simulink model "Excavator_Motion"  (R2026a)
settings: Solver=ode23t  StopTime=activeTestPos.getElement('swingAng').Time(end)  MaxStep=0.1  AbsTol=1e-3
PostLoadFcn:
  | set_param(bdroot,'IgnoredZcDiagnostic','none');
  | activeTestPos = ScenarioMotion.loadedBucketDigCycle;
model workspace: external: MAT-File ExcavatorAssemblyDataStruct.mat (data not in the file)
undefined symbols (not defined in the file or in its folder): Bo, Bu, gravity, materialWeight, P28Assembly, startDiggingZPos, velocityToYForceGain, X, Y, yForceMax, yForceToZForceGain, Z, zForceMax
libraries: sm_lib x79, nesl_utility x41, Excavator_Parts_Lib x8, simulink x2, simulink_extras x1
(part 1 of 3)
Description:
  | Excavator with Actuator Force Calculation
  | 
  | Copyright 2022-2026 The MathWorks, Inc.
settings Model: Creator=gabri  LastModifiedBy=smiller
settings SolverCC: MaxConsecutiveMinStep=10  ZeroCrossAlgorithm=Adaptive  DecoupledContinuousIntegration=on  MinimalZcImpactIntegration=on
settings DataIOCC: ExternalInput=activeTestPos  LoadExternalInput=on  SignalLoggingName=logsout_Excavator_Motion  ReturnWorkspaceOutputsName=simOut
settings DebuggingCC: IgnoredZcDiagnostic=none
settings SimscapeCC: SimscapeNominalValues="[{\"value\":\"1\",\"unit\":\"A\"},{\"value\":\"1\",\"unit\":\"bar\"},{\"value\":\"1\",\"unit\":\"cm^2\"},{\"value\":\"1\",\"unit\":\"cm^3/s\"},{\"value\":\"1\",\"unit\":\"kJ/kg\"},{\"value\":\"1\",\"unit\":\"kW\"},{\"value\":\"1\",\"unit\":\"l\"},{\"value\":\"1\",\"unit\":\"N\"},{\"value\":\"1\",\"unit\":\"N*m\"},{\"value\":\"1\",\"unit\":\"V\"}]"  SimscapeLogName=simlog_Excavator_Motion  SimscapeLogLimitData=off  SimscapeLogDataHistory=5000.0
settings DiagnosticsConfigSet: SimMechanicsConflictingReferenceFrames=none
settings ExplorerConfigSet: InternalSimMechanicsExplorerSettings="<ExplorerConfiguration><canonicalview>default</canonicalview><AnimationSetting><BasePlaybackSpeed>1.0</BasePlaybackSpeed><PlaybackSpeedFactor>1.0</PlaybackSpeedFactor></AnimationSetting><TilePanel><TileInfo><Tiles Columns=\"1\" Count=\"1\" Rows=\"1\"><Column Weight=\"1\"/><Row Weight=\"1\"/><Tile Height=\"1\" Width=\"1\" X=\"0\" Y=\"0\"/></Tiles></TileInfo><SceneInfo><SceneViewer><BGColor><R>1</R><G>1</G><B>1</B></BGColor><Camera><DoPerspective>off</DoPerspective><Position><X>27.5807103687801352</X><Y>37.4081583974126985</Y><Z>9.98244775872054291</Z></Position><Center><X>8.99598322856128263</X><Y>12.20284550619599</Y><Z>4.4342740611865441</Z></Center><Up><X>-0.106919570484384385</X><Y>-0.137906585416309235</Y><Z>0.984657290201138458</Z></Up><ViewLimDist>1</ViewLimDist><YLim>6.11731328526511131</YLim><XLim>12.9452235683135441</XLim></Camera></SceneViewer></SceneInfo></TilePanel><MechEditorPanel><Cameras/><GfxPanelCameraMap/><VideoCreator><PlaybackSpeedRatio>1.0</PlaybackSpeedRatio><FrameRate>30</FrameRate><VideoFormat>Motion JPEG AVI</VideoFormat><FrameSize>auto</FrameSize></VideoCreator></MechEditorPanel></ExplorerConfiguration>"

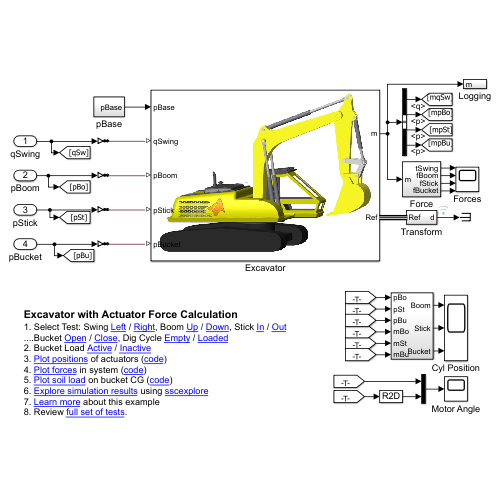
[thumbnail: Simulink's stored preview of the top-level diagram]
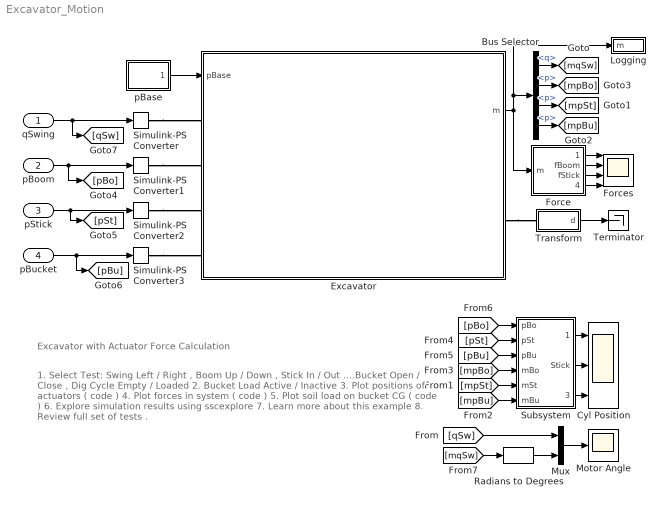
== system Excavator_Motion ==
  note: Excavator with Actuator Force Calculation
  note: 1. Select Test: Swing Left / Right , Boom Up / Down , Stick In / Out
      | ....Bucket Open / Close , Dig Cycle Empty / Loaded
      | 2. Bucket Load Active / Inactive
      | 3. Plot positions of actuators ( code )
      | 4. Plot forces in system ( code )
      | 5. Plot soil load on bucket CG ( code )
      | 6. Explore simulation results using sscexplore
      | 7. Learn more about this example
      | 8. Review full set of tests .
  qSwing : Inport
  pBoom : Inport  Port=2
  pStick : Inport  Port=3
  pBucket : Inport  Port=4
  Bus Selector : BusSelector  OutputSignals=Swing.q,Boom.p,Stick.p,Bucket.p
  Cyl Position : Scope  NumInputPorts=3
      settings: ActiveDisplayYMinimum=-0.10545  ActiveDisplayYMaximum=1.26585
  Excavator : Subsystem
      mask Display: image('Excavator_CAD_Full_IMAGE.png');
  Force : Subsystem
  Forces : Scope  NumInputPorts=4
      settings: ActiveDisplayYMinimum=-530.22843  ActiveDisplayYMaximum=1858.3528  DataLoggingVariableName=ScopeData2
  Logging : Subsystem
  Motor Angle : Scope
      settings: ActiveDisplayYMinimum=-135.21911  ActiveDisplayYMaximum=16.97108
  Mux : Mux  Inputs=2
  Radians to Degrees : simulink_extras/Transformations/Radians to Degrees
  Simulink-PS Converter : nesl_utility/Simulink-PS Converter  PhysicalDomain=network_engine_domain  SubClassName=ps_input  LeftPortType=input  RightPortType=output  PseudoPeriodic=off  Frequencies=[]  NoiseDistribution=none  NoiseParameters=[]  Unit=deg  AffineConversion=off  FilteringAndDerivatives=filter  SimscapeFilterOrder=2  InputFilterTimeConstant=0.05  UdotUserProvided=0
  Simulink-PS Converter1 : nesl_utility/Simulink-PS Converter  PhysicalDomain=network_engine_domain  SubClassName=ps_input  LeftPortType=input  RightPortType=output  PseudoPeriodic=off  Frequencies=[]  NoiseDistribution=none  NoiseParameters=[]  Unit=mm  AffineConversion=off  FilteringAndDerivatives=filter  SimscapeFilterOrder=2  InputFilterTimeConstant=0.05  UdotUserProvided=0
  Simulink-PS Converter2 : nesl_utility/Simulink-PS Converter  PhysicalDomain=network_engine_domain  SubClassName=ps_input  LeftPortType=input  RightPortType=output  PseudoPeriodic=off  Frequencies=[]  NoiseDistribution=none  NoiseParameters=[]  Unit=mm  AffineConversion=off  FilteringAndDerivatives=filter  SimscapeFilterOrder=2  InputFilterTimeConstant=0.05  UdotUserProvided=0
  Simulink-PS Converter3 : nesl_utility/Simulink-PS Converter  PhysicalDomain=network_engine_domain  SubClassName=ps_input  LeftPortType=input  RightPortType=output  PseudoPeriodic=off  Frequencies=[]  NoiseDistribution=none  NoiseParameters=[]  Unit=mm  AffineConversion=off  FilteringAndDerivatives=filter  SimscapeFilterOrder=2  InputFilterTimeConstant=0.05  UdotUserProvided=0
  Subsystem : Subsystem
  Terminator : Terminator
  Transform : Subsystem
  pBase : Subsystem
  wires:
  pBoom/1 -> Simulink-PS Converter1/1, [pBo]
  pStick/1 -> Simulink-PS Converter2/1, [pSt]
  qSwing/1 -> [qSw], Simulink-PS Converter/1
  pBucket/1 -> [pBu], Simulink-PS Converter3/1
  Excavator/1(m) -> Bus Selector/1, Logging/1(m), Force/1(m)
  Bus Selector/1 -> [mqSw]  "<q>"
  Bus Selector/2 -> [mpBo]  "<p>"
  Bus Selector/3 -> [mpSt]  "<p>"
  Bus Selector/4 -> [mpBu]  "<p>"
  [mpBo] -> Subsystem/4(mBo)
  [mpSt] -> Subsystem/5(mSt)
  [mpBu] -> Subsystem/6(mBu)
  Subsystem/1(Boom) -> Cyl Position/1
  Subsystem/2(Stick) -> Cyl Position/2
  Subsystem/3(Bucket) -> Cyl Position/3
  [pBo] -> Subsystem/1(pBo)
  [pSt] -> Subsystem/2(pSt)
  [pBu] -> Subsystem/3(pBu)
  [qSw] -> Mux/1
  [mqSw] -> Radians to Degrees/1
  Mux/1 -> Motor Angle/1
  Radians to Degrees/1 -> Mux/2
  Force/1(tSwing) -> Forces/1
  Force/2(fBoom) -> Forces/2
  Force/3(fStick) -> Forces/3
  Force/4(fBucket) -> Forces/4
  Transform/1(d) -> Terminator/1
  pBase/1(pBase) -> Excavator/1(pBase)
  connections:
  Simulink-PS Converter/RConn1 -- Excavator/LConn1
  Simulink-PS Converter1/RConn1 -- Excavator/LConn2
  Simulink-PS Converter2/RConn1 -- Excavator/LConn3
  Simulink-PS Converter3/RConn1 -- Excavator/LConn4
  Excavator/RConn1 -- Transform/LConn1

== system Excavator_Motion/Excavator ==
  pBase : Inport
  Machine : Subsystem
      mask Display: image('Excavator_CAD_Full_IMAGE.png');
  qSwing : PMIOPort  Side=Left
  pBoom : PMIOPort  Port=2  Side=Left
  pStick : PMIOPort  Port=3  Side=Left
  pBucket : PMIOPort  Port=4  Side=Left
  Ref : PMIOPort  Port=5  Side=Right
  m : Outport
  wires:
  Machine/1(m) -> m/1
  pBase/1 -> Machine/1(pBase)
  connections:
  qSwing/RConn1 -- Machine/LConn1
  pBoom/RConn1 -- Machine/LConn2
  pStick/RConn1 -- Machine/LConn3
  pBucket/RConn1 -- Machine/LConn4
  Machine/RConn1 -- Ref/RConn1

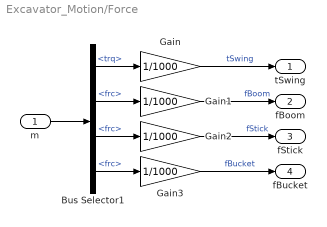
== system Excavator_Motion/Force ==
  m : Inport
  Bus Selector1 : BusSelector  OutputSignals=Swing.trq,Boom.frc,Stick.frc,Bucket.frc
  Gain{,1..3} (4 alike) : Gain  Gain=1/1000
  tSwing : Outport
  fBoom : Outport  Port=2
  fStick : Outport  Port=3
  fBucket : Outport  Port=4
  wires:
  Bus Selector1/1 -> Gain/1  "<trq>"
  Bus Selector1/2 -> Gain1/1  "<frc>"
  m/1 -> Bus Selector1/1
  Bus Selector1/3 -> Gain2/1  "<frc>"
  Bus Selector1/4 -> Gain3/1  "<frc>"
  Gain/1 -> tSwing/1  "tSwing"
  Gain1/1 -> fBoom/1  "fBoom"
  Gain2/1 -> fStick/1  "fStick"
  Gain3/1 -> fBucket/1  "fBucket"

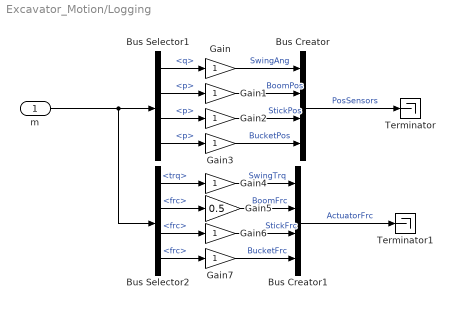
== system Excavator_Motion/Logging ==
  m : Inport
  Bus Creator : BusCreator  Inputs=4
  Bus Creator1 : BusCreator  Inputs=4
  Bus Selector1 : BusSelector  OutputSignals=Swing.q,Boom.p,Stick.p,Bucket.p
  Bus Selector2 : BusSelector  OutputSignals=Swing.trq,Boom.frc,Stick.frc,Bucket.frc
  Gain{,1..4,6..7} (7 alike) : Gain
  Gain5 : Gain  Gain=0.5
  Terminator : Terminator
  Terminator1 : Terminator
  wires:
  m/1 -> Bus Selector2/1, Bus Selector1/1
  Bus Selector1/1 -> Gain/1  "<q>"
  Bus Selector1/2 -> Gain1/1  "<p>"
  Bus Selector1/3 -> Gain2/1  "<p>"
  Bus Selector1/4 -> Gain3/1  "<p>"
  Gain/1 -> Bus Creator/1  "SwingAng"
  Gain1/1 -> Bus Creator/2  "BoomPos"
  Gain2/1 -> Bus Creator/3  "StickPos"
  Gain3/1 -> Bus Creator/4  "BucketPos"
  Bus Creator/1 -> Terminator/1  "PosSensors"
  Bus Selector2/4 -> Gain7/1  "<frc>"
  Bus Selector2/3 -> Gain6/1  "<frc>"
  Bus Selector2/2 -> Gain5/1  "<frc>"
  Bus Selector2/1 -> Gain4/1  "<trq>"
  Bus Creator1/1 -> Terminator1/1  "ActuatorFrc"
  Gain7/1 -> Bus Creator1/4  "BucketFrc"
  Gain6/1 -> Bus Creator1/3  "StickFrc"
  Gain5/1 -> Bus Creator1/2  "BoomFrc"
  Gain4/1 -> Bus Creator1/1  "SwingTrq"

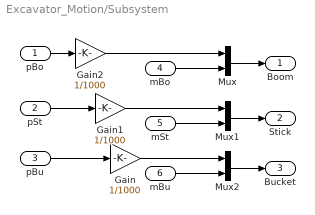
== system Excavator_Motion/Subsystem ==
  pBo : Inport
  pSt : Inport  Port=2
  pBu : Inport  Port=3
  mBo : Inport  Port=4
  mSt : Inport  Port=5
  mBu : Inport  Port=6
  Gain : Gain  Gain=1/1000
  Gain1 : Gain  Gain=1/1000
  Gain2 : Gain  Gain=1/1000
  Mux : Mux  Inputs=2
  Mux1 : Mux  Inputs=2
  Mux2 : Mux  Inputs=2
  Boom : Outport
  Stick : Outport  Port=2
  Bucket : Outport  Port=3
  wires:
  Mux1/1 -> Stick/1
  Mux/1 -> Boom/1
  Mux2/1 -> Bucket/1
  Gain/1 -> Mux2/1
  Gain2/1 -> Mux/1
  pBo/1 -> Gain2/1
  Gain1/1 -> Mux1/1
  pBu/1 -> Gain/1
  mBo/1 -> Mux/2
  pSt/1 -> Gain1/1
  mSt/1 -> Mux1/2
  mBu/1 -> Mux2/2

== system Excavator_Motion/Transform ==
  Part Pos Ori : Excavator_Parts_Lib/Part Pos Ori  SystemSampleTime=-1  VariantActivationTime=update diagram  EmptyChoice=off  PassThrough=off  PassThroughVariantControl=(default)  EmptyChoiceVariantControl=(default)  AllowFlexibleInterface=on  Latency=0  AutoFrameSizeCalculation=off
  Part Pos Ori1 : Excavator_Parts_Lib/Part Pos Ori  SystemSampleTime=-1  VariantActivationTime=update diagram  EmptyChoice=off  PassThrough=off  PassThroughVariantControl=(default)  EmptyChoiceVariantControl=(default)  AllowFlexibleInterface=on  Latency=0  AutoFrameSizeCalculation=off
  Simscape Bus : SimscapeBus  HierarchyStrings=Bo;Bu
  Ref : PMIOPort  Side=Left
  Out Bus Element : Outport  PortName=d  Element=Boom
  Out Bus Element1 : Outport  PortName=d  Element=Bucket
  wires:
  Part Pos Ori1/1 -> Out Bus Element/1
  Part Pos Ori/1 -> Out Bus Element1/1
  connections:
  Ref/RConn1 -- Simscape Bus/RConn1
  Part Pos Ori1/LConn1 -- Simscape Bus/LConn1
  Part Pos Ori/LConn1 -- Simscape Bus/LConn2

== system Excavator_Motion/pBase ==
  Bus Creator : BusCreator  Inputs=3
  Constant : Constant  Value=0
  Constant1 : Constant  Value=0
  Constant2 : Constant  Value=0
  pBase : Outport
  wires:
  Bus Creator/1 -> pBase/1
  Constant/1 -> Bus Creator/1  "px"
  Constant1/1 -> Bus Creator/2  "py"
  Constant2/1 -> Bus Creator/3  "qz"

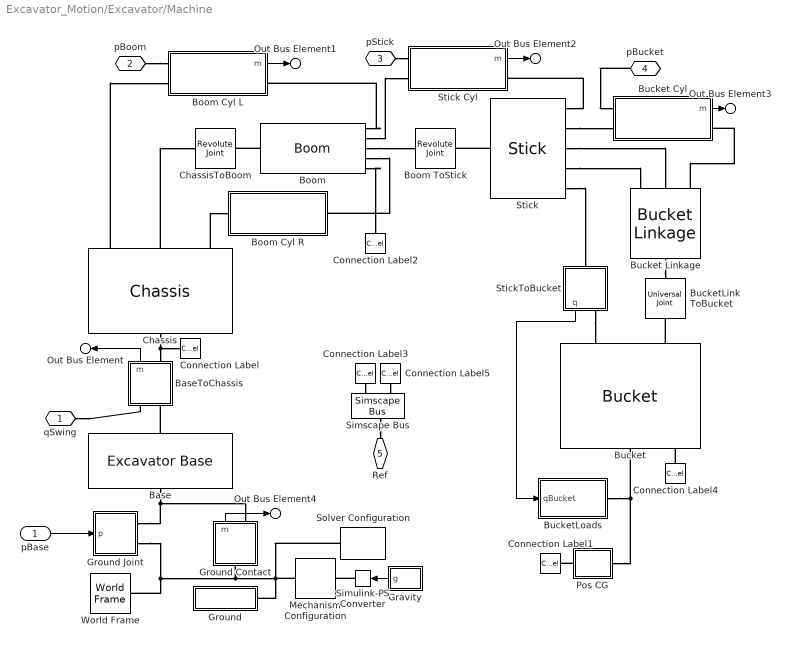
== system Excavator_Motion/Excavator/Machine ==
  pBase : Inport
  Base : Excavator_Parts_Lib/Excavator Base  Tag=AAA55596-1DB0-4345-9724-6685E48489E2
  BaseToChassis : Subsystem  Tag=1fdcb50d-bed1-4557-9df5-71c57fded59e
      mask Display: image('Excavator_Revolute_IMAGE.png')
  Boom : Excavator_Parts_Lib/Boom  Tag=FF941BC7-23B6-8A4E-AE2C-D7583C913694  opc=1  part_clr=excv_data.arm.clr
  Boom ToStick : sm_lib/Joints/Revolute Joint  JointMode=Normal  CompositeWrenchDir=FollowerOnBase  CompositeWrenchFrame=BaseFrame  SenseConstraintForce=off  SenseConstraintTorque=off  SenseTotalForce=off  SenseTotalTorque=off  PositionTargetSpecify=on  PositionTargetPriority=Low  PositionTargetValue=initBoomToStickRevPos  PositionTargetValueUnits=deg  VelocityTargetSpecify=off  VelocityTargetPriority=High  VelocityTargetValue=0  VelocityTargetValueUnits=deg/s  EquilibriumPosition=0  EquilibriumPositionUnits=deg  SpringStiffness=0  SpringStiffnessUnits=N*m/deg  DampingCoefficient=0  DampingCoefficientUnits=N*m/(deg/s)  LowerLimitSpecify=off  LowerLimitBound=-90  LowerLimitBoundUnits=deg  LowerLimitStiffness=1e4  LowerLimitStiffnessUnits=N*m/deg  LowerLimitDamping=10  LowerLimitDampingUnits=N*m/(deg/s)  LowerLimitTransitionRegionWidth=0.1  LowerLimitTransitionRegionWidthUnits=deg  UpperLimitSpecify=off  UpperLimitBound=90  UpperLimitBoundUnits=deg  UpperLimitStiffness=1e4  UpperLimitStiffnessUnits=N*m/deg  UpperLimitDamping=10  UpperLimitDampingUnits=N*m/(deg/s)  UpperLimitTransitionRegionWidth=0.1  UpperLimitTransitionRegionWidthUnits=deg  TorqueActuationMode=NoTorque  MotionActuationMode=ComputedMotion  SensePosition=off  SenseVelocity=off  SenseAcceleration=off  SenseTorqueForce=off  SenseLowerLimitTorqueForce=off  SenseUpperLimitTorqueForce=off
  Boom Cyl L : Subsystem
      mask Display: image('Excavator_Cylinder_Actuate_IMAGE.png')
  Boom Cyl R : Subsystem
      mask Display: image('Excavator_Cylinder_Actuate_IMAGE.png')
  Bucket : Excavator_Parts_Lib/Bucket  Tag=FF47B028-216B-7042-A7FD-934F60E6CEA6  opc=1  part_clr=excv_data.arm.clr
  Bucket Linkage : Excavator_Parts_Lib/Bucket Linkage
  Bucket Cyl : Subsystem
      mask Display: image('Excavator_Cylinder_Actuate_IMAGE.png')
  BucketLink ToBucket : sm_lib/Joints/Universal Joint  JointMode=Normal  CompositeWrenchDir=FollowerOnBase  CompositeWrenchFrame=BaseFrame  SenseConstraintForce=off  SenseConstraintTorque=off  SenseTotalForce=off  SenseTotalTorque=off  RxPositionTargetSpecify=on  RxPositionTargetPriority=Low  RxPositionTargetValue=-10  RxPositionTargetValueUnits=deg  RxVelocityTargetSpecify=off  RxVelocityTargetPriority=High  RxVelocityTargetValue=0  RxVelocityTargetValueUnits=deg/s  RxEquilibriumPosition=0  RxEquilibriumPositionUnits=deg  RxSpringStiffness=0  RxSpringStiffnessUnits=N*m/deg  RxDampingCoefficient=0  RxDampingCoefficientUnits=N*m/(deg/s)  RxLowerLimitSpecify=off  RxLowerLimitBound=-90  RxLowerLimitBoundUnits=deg  RxLowerLimitStiffness=1e4  RxLowerLimitStiffnessUnits=N*m/deg  RxLowerLimitDamping=10  RxLowerLimitDampingUnits=N*m/(deg/s)  RxLowerLimitTransitionRegionWidth=0.1  RxLowerLimitTransitionRegionWidthUnits=deg  RxUpperLimitSpecify=off  RxUpperLimitBound=90  RxUpperLimitBoundUnits=deg  RxUpperLimitStiffness=1e4  RxUpperLimitStiffnessUnits=N*m/deg  RxUpperLimitDamping=10  RxUpperLimitDampingUnits=N*m/(deg/s)  RxUpperLimitTransitionRegionWidth=0.1  RxUpperLimitTransitionRegionWidthUnits=deg  RxTorqueActuationMode=NoTorque  RxMotionActuationMode=ComputedMotion  RxSensePosition=off  RxSenseVelocity=off  RxSenseAcceleration=off  RxSenseTorqueForce=off  RxSenseLowerLimitTorqueForce=off  RxSenseUpperLimitTorqueForce=off  RyPositionTargetSpecify=on  RyPositionTargetPriority=High  RyPositionTargetValue=0  RyPositionTargetValueUnits=deg  RyVelocityTargetSpecify=off  RyVelocityTargetPriority=High  RyVelocityTargetValue=0  RyVelocityTargetValueUnits=deg/s  RyEquilibriumPosition=0  RyEquilibriumPositionUnits=deg  RySpringStiffness=0  RySpringStiffnessUnits=N*m/deg  RyDampingCoefficient=0  RyDampingCoefficientUnits=N*m/(deg/s)  RyLowerLimitSpecify=off  RyLowerLimitBound=-90  RyLowerLimitBoundUnits=deg  RyLowerLimitStiffness=1e4  RyLowerLimitStiffnessUnits=N*m/deg  RyLowerLimitDamping=10  RyLowerLimitDampingUnits=N*m/(deg/s)  RyLowerLimitTransitionRegionWidth=0.1  RyLowerLimitTransitionRegionWidthUnits=deg  RyUpperLimitSpecify=off  RyUpperLimitBound=90  RyUpperLimitBoundUnits=deg  RyUpperLimitStiffness=1e4  RyUpperLimitStiffnessUnits=N*m/deg  RyUpperLimitDamping=10  RyUpperLimitDampingUnits=N*m/(deg/s)  RyUpperLimitTransitionRegionWidth=0.1  RyUpperLimitTransitionRegionWidthUnits=deg  RyTorqueActuationMode=NoTorque  RyMotionActuationMode=ComputedMotion  RySensePosition=off  RySenseVelocity=off  RySenseAcceleration=off  RySenseTorqueForce=off  RySenseLowerLimitTorqueForce=off  RySenseUpperLimitTorqueForce=off
  BucketLoads : Subsystem
  Chassis : Excavator_Parts_Lib/Chassis  Tag=19F311DB-9E7A-8F4D-82CB-D8DCD5D4899B  opc=1
  ChassisToBoom : sm_lib/Joints/Revolute Joint  JointMode=Normal  CompositeWrenchDir=FollowerOnBase  CompositeWrenchFrame=BaseFrame  SenseConstraintForce=off  SenseConstraintTorque=off  SenseTotalForce=off  SenseTotalTorque=off  PositionTargetSpecify=on  PositionTargetPriority=Low  PositionTargetValue=initChassisToBoomRevPos  PositionTargetValueUnits=deg  VelocityTargetSpecify=off  VelocityTargetPriority=High  VelocityTargetValue=0  VelocityTargetValueUnits=deg/s  EquilibriumPosition=0  EquilibriumPositionUnits=deg  SpringStiffness=0  SpringStiffnessUnits=N*m/deg  DampingCoefficient=0  DampingCoefficientUnits=N*m/(deg/s)  LowerLimitSpecify=off  LowerLimitBound=-90  LowerLimitBoundUnits=deg  LowerLimitStiffness=1e4  LowerLimitStiffnessUnits=N*m/deg  LowerLimitDamping=10  LowerLimitDampingUnits=N*m/(deg/s)  LowerLimitTransitionRegionWidth=0.1  LowerLimitTransitionRegionWidthUnits=deg  UpperLimitSpecify=off  UpperLimitBound=90  UpperLimitBoundUnits=deg  UpperLimitStiffness=1e4  UpperLimitStiffnessUnits=N*m/deg  UpperLimitDamping=10  UpperLimitDampingUnits=N*m/(deg/s)  UpperLimitTransitionRegionWidth=0.1  UpperLimitTransitionRegionWidthUnits=deg  TorqueActuationMode=NoTorque  MotionActuationMode=ComputedMotion  SensePosition=off  SenseVelocity=off  SenseAcceleration=off  SenseTorqueForce=off  SenseLowerLimitTorqueForce=off  SenseUpperLimitTorqueForce=off
  Connection Label : ConnectionLabel  Label=Cha
  Connection Label1 : ConnectionLabel  Label=Cha
  Connection Label2 : ConnectionLabel  Label=Bo
  Connection Label3 : ConnectionLabel  Label=Bo
  Connection Label4 : ConnectionLabel  Label=Bu
  Connection Label5 : ConnectionLabel  Label=Bu
  Gravity : Subsystem
  Ground : Subsystem
  Ground Contact : Subsystem
  Ground Joint : Subsystem
  Mechanism Configuration : sm_lib/Utilities/Mechanism Configuration  UniformGravity=TimeVarying  GravityVector=[0 0 -9.80665]  GravityVectorUnits=m/s^2  LinearizationDelta=0.001  JointModeTransitionNonlinearIterations=2
  Pos CG : Subsystem
  Simscape Bus : SimscapeBus  HierarchyStrings=Bo;Bu
  Simulink-PS Converter : nesl_utility/Simulink-PS Converter  PhysicalDomain=network_engine_domain  SubClassName=ps_input  LeftPortType=input  RightPortType=output  PseudoPeriodic=off  Frequencies=[]  NoiseDistribution=none  NoiseParameters=[]  Unit=m/s^2  AffineConversion=off  FilteringAndDerivatives=provide  SimscapeFilterOrder=1  InputFilterTimeConstant=0.001  UdotUserProvided=0
  Solver Configuration : nesl_utility/Solver Configuration  PhysicalDomain=network_engine_domain  SubClassName=solver  LeftPortType=input  RightPortType=generic  Tones=[]  Harmonics=[]  SimulateNoise=off  Profile=off  UseLocalSampling=off  EnableSwitchedLinearOptims=on  FrequencyDomain=off  UseCCode=off  RelTol=0.001  AbsTol=0.001  MinStep=1e-09  ToWorkspace=off  RevertToSquareIcSolve=off  NumHomotopyIterations=100  PhasorMode=off  PhasorModeNumHarmonics=1  ConsistencySolver=NEWTON_XTOL_AFTER_FTOL  CanonicalOrdering=UNORDERED  OptimizeIntermediates=UNOPTIMIZED  IndexReductionMethod=DerivativeReplacement  DoDC=off  ResidualTolerance=1e-09  ConsistencyTolSource=GLOBAL  ConsistencyAbsTol=0.001  ConsistencyRelTol=0.001  ConsistencyTolFactor=0.001  UseLocalSolver=off  LocalSolverChoice=NE_BACKWARD_EULER_ADVANCER  ResolveIndetEquations=on  FunctionEvalNumThread=1  LocalSolverSampleTime=0.001  DoFixedCost=off  MaxNonlinIter=3  MaxModeIter=2  ComputeImpulses=off  ImpulseIterations=2  LinearAlgebra=auto  LinearAlgebraNumThread=0  EquationFormulation=NE_TIME_EF  DelaysMemoryBudget=1024  AutomaticFiltering=on  FilteringTimeConstant=0.001  PartitionStorageMethod=AS_NEEDED  PartitionMemoryBudget=1024  PartitionMethod=ROBUST  MultibodyUseLocalSolver=off  MultibodyLocalSolverChoice=ODE1  MultibodyLocalSolverSampleTime=0.001
  Stick : Excavator_Parts_Lib/Stick  Tag=62A93771-C790-5E4F-BFD2-96C4D317E04B  opc=1  part_clr=excv_data.arm.clr
  Stick Cyl : Subsystem
      mask Display: image('Excavator_Cylinder_Actuate_IMAGE.png')
  StickToBucket : Subsystem  Tag=07adba86-714b-4e09-8ef8-8682a71cd5e3
      mask Display: image('Excavator_Revolute_IMAGE.png')
  World Frame : sm_lib/Frames and Transforms/World Frame
  qSwing : PMIOPort  Side=Left
  pBoom : PMIOPort  Port=2  Side=Left
  pStick : PMIOPort  Port=3  Side=Left
  pBucket : PMIOPort  Port=4  Side=Left
  Ref : PMIOPort  Port=5  Side=Right
  Out Bus Element : Outport  PortName=m  Element=Swing
  Out Bus Element1 : Outport  PortName=m  Element=Boom
  Out Bus Element2 : Outport  PortName=m  Element=Stick
  Out Bus Element3 : Outport  PortName=m  Element=Bucket
  Out Bus Element4 : Outport  PortName=m  Element=frcGround
  wires:
  Gravity/1(g) -> Simulink-PS Converter/1
  BaseToChassis/1(m) -> Out Bus Element/1
  Boom Cyl L/1(m) -> Out Bus Element1/1
  Stick Cyl/1(m) -> Out Bus Element2/1
  Bucket Cyl/1(m) -> Out Bus Element3/1
  StickToBucket/1(q) -> BucketLoads/1(qBucket)
  Ground Contact/1(m) -> Out Bus Element4/1
  pBase/1 -> Ground Joint/1(p)
  connections:
  Chassis/LConn1 -- Connection Label/LConn1 -- BaseToChassis/RConn1
  Base/RConn1 -- BaseToChassis/LConn2
  Chassis/RConn2 -- ChassisToBoom/LConn1
  Boom/RConn3 -- Boom ToStick/LConn1
  Stick/RConn5 -- StickToBucket/LConn1
  StickToBucket/RConn1 -- Bucket/LConn1
  Stick/RConn2 -- Bucket Cyl/LConn2
  Stick/RConn4 -- Bucket Linkage/LConn1
  Stick/RConn3 -- Bucket Linkage/LConn2
  Simulink-PS Converter/RConn1 -- Mechanism Configuration/LConn1
  Mechanism Configuration/RConn1 -- Solver Configuration/RConn1 -- Ground Joint/RConn2 -- World Frame/RConn1 -- Ground Contact/LConn1 -- Ground/LConn1
  Boom/LConn1 -- ChassisToBoom/RConn1
  Boom/RConn2 -- Stick Cyl/LConn2
  Bucket/LConn2 -- BucketLink ToBucket/RConn1
  Bucket Linkage/RConn1 -- BucketLink ToBucket/LConn1
  Pos CG/RConn1 -- BucketLoads/RConn1 -- Bucket/RConn2
  Boom/RConn1 -- Boom Cyl L/RConn1
  Chassis/RConn1 -- Boom Cyl L/LConn2
  Chassis/RConn3 -- Boom Cyl R/LConn1
  Boom/RConn4 -- Boom Cyl R/RConn1
  Stick/RConn1 -- Stick Cyl/RConn1
  Stick/LConn1 -- Boom ToStick/RConn1
  Bucket Linkage/LConn3 -- Bucket Cyl/RConn1
  Pos CG/LConn1 -- Connection Label1/LConn1
  pBoom/RConn1 -- Boom Cyl L/LConn1
  qSwing/RConn1 -- BaseToChassis/LConn1
  pStick/RConn1 -- Stick Cyl/LConn1
  pBucket/RConn1 -- Bucket Cyl/LConn1
  Boom/RConn5 -- Connection Label2/LConn1
  Connection Label3/LConn1 -- Simscape Bus/LConn1
  Simscape Bus/RConn1 -- Ref/RConn1
  Base/LConn1 -- Ground Contact/RConn1 -- Ground Joint/RConn1
  Connection Label4/LConn1 -- Bucket/RConn3
  Connection Label5/LConn1 -- Simscape Bus/LConn2

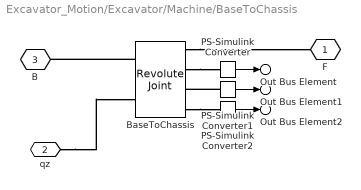
== system Excavator_Motion/Excavator/Machine/BaseToChassis ==
  BaseToChassis : sm_lib/Joints/Revolute Joint  JointMode=Normal  CompositeWrenchDir=FollowerOnBase  CompositeWrenchFrame=BaseFrame  SenseConstraintForce=off  SenseConstraintTorque=off  SenseTotalForce=off  SenseTotalTorque=off  PositionTargetSpecify=on  PositionTargetPriority=High  PositionTargetValue=activeTestPos.getElement('swingAng').Data(1)  PositionTargetValueUnits=deg  VelocityTargetSpecify=on  VelocityTargetPriority=High  VelocityTargetValue=0  VelocityTargetValueUnits=deg/s  EquilibriumPosition=0  EquilibriumPositionUnits=deg  SpringStiffness=0  SpringStiffnessUnits=N*m/deg  DampingCoefficient=0  DampingCoefficientUnits=N*m/(deg/s)  LowerLimitSpecify=off  LowerLimitBound=-90  LowerLimitBoundUnits=deg  LowerLimitStiffness=1e4  LowerLimitStiffnessUnits=N*m/deg  LowerLimitDamping=10  LowerLimitDampingUnits=N*m/(deg/s)  LowerLimitTransitionRegionWidth=0.1  LowerLimitTransitionRegionWidthUnits=deg  UpperLimitSpecify=off  UpperLimitBound=90  UpperLimitBoundUnits=deg  UpperLimitStiffness=1e4  UpperLimitStiffnessUnits=N*m/deg  UpperLimitDamping=10  UpperLimitDampingUnits=N*m/(deg/s)  UpperLimitTransitionRegionWidth=0.1  UpperLimitTransitionRegionWidthUnits=deg  TorqueActuationMode=ComputedTorque  MotionActuationMode=InputMotion  SensePosition=on  SenseVelocity=on  SenseAcceleration=off  SenseTorqueForce=on  SenseLowerLimitTorqueForce=off  SenseUpperLimitTorqueForce=off
  PS-Simulink Converter : nesl_utility/PS-Simulink Converter  PhysicalDomain=network_engine_domain  SubClassName=ps_output  LeftPortType=input  RightPortType=output  PseudoPeriodic=off  Frequencies=[]  VectorFormat=inherit  Unit=rad  AffineConversion=off
  PS-Simulink Converter1 : nesl_utility/PS-Simulink Converter  PhysicalDomain=network_engine_domain  SubClassName=ps_output  LeftPortType=input  RightPortType=output  PseudoPeriodic=off  Frequencies=[]  VectorFormat=inherit  Unit=rad/s  AffineConversion=off
  PS-Simulink Converter2 : nesl_utility/PS-Simulink Converter  PhysicalDomain=network_engine_domain  SubClassName=ps_output  LeftPortType=input  RightPortType=output  PseudoPeriodic=off  Frequencies=[]  VectorFormat=inherit  Unit=N*m  AffineConversion=off
  F : PMIOPort  Side=Right
  qz : PMIOPort  Port=2  Side=Left
  B : PMIOPort  Port=3  Side=Left
  Out Bus Element : Outport  PortName=m  Element=q
  Out Bus Element1 : Outport  PortName=m  Element=w
  Out Bus Element2 : Outport  PortName=m  Element=trq
  wires:
  PS-Simulink Converter/1 -> Out Bus Element/1
  PS-Simulink Converter1/1 -> Out Bus Element1/1
  PS-Simulink Converter2/1 -> Out Bus Element2/1
  connections:
  BaseToChassis/RConn1 -- F/RConn1
  BaseToChassis/LConn1 -- B/RConn1
  qz/RConn1 -- BaseToChassis/LConn2
  BaseToChassis/RConn2 -- PS-Simulink Converter/LConn1
  PS-Simulink Converter1/LConn1 -- BaseToChassis/RConn3
  BaseToChassis/RConn4 -- PS-Simulink Converter2/LConn1

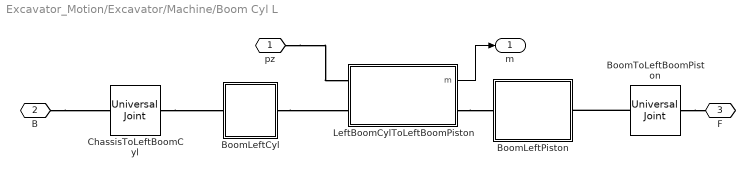
== system Excavator_Motion/Excavator/Machine/Boom Cyl L ==
  BoomLeftCyl : Subsystem  Tag=4F70B330-6F24-E84C-8BE5-4F108E58AE93
  BoomLeftPiston : Subsystem  Tag=45215E48-B489-9D47-85FC-0A495393BD12
  BoomToLeftBoomPiston : sm_lib/Joints/Universal Joint  JointMode=Normal  CompositeWrenchDir=FollowerOnBase  CompositeWrenchFrame=BaseFrame  SenseConstraintForce=off  SenseConstraintTorque=off  SenseTotalForce=off  SenseTotalTorque=off  RxPositionTargetSpecify=off  RxPositionTargetPriority=High  RxPositionTargetValue=0  RxPositionTargetValueUnits=deg  RxVelocityTargetSpecify=off  RxVelocityTargetPriority=High  RxVelocityTargetValue=0  RxVelocityTargetValueUnits=deg/s  RxEquilibriumPosition=0  RxEquilibriumPositionUnits=deg  RxSpringStiffness=0  RxSpringStiffnessUnits=N*m/deg  RxDampingCoefficient=0  RxDampingCoefficientUnits=N*m/(deg/s)  RxLowerLimitSpecify=off  RxLowerLimitBound=-90  RxLowerLimitBoundUnits=deg  RxLowerLimitStiffness=1e4  RxLowerLimitStiffnessUnits=N*m/deg  RxLowerLimitDamping=10  RxLowerLimitDampingUnits=N*m/(deg/s)  RxLowerLimitTransitionRegionWidth=0.1  RxLowerLimitTransitionRegionWidthUnits=deg  RxUpperLimitSpecify=off  RxUpperLimitBound=90  RxUpperLimitBoundUnits=deg  RxUpperLimitStiffness=1e4  RxUpperLimitStiffnessUnits=N*m/deg  RxUpperLimitDamping=10  RxUpperLimitDampingUnits=N*m/(deg/s)  RxUpperLimitTransitionRegionWidth=0.1  RxUpperLimitTransitionRegionWidthUnits=deg  RxTorqueActuationMode=NoTorque  RxMotionActuationMode=ComputedMotion  RxSensePosition=off  RxSenseVelocity=off  RxSenseAcceleration=off  RxSenseTorqueForce=off  RxSenseLowerLimitTorqueForce=off  RxSenseUpperLimitTorqueForce=off  RyPositionTargetSpecify=off  RyPositionTargetPriority=High  RyPositionTargetValue=0  RyPositionTargetValueUnits=deg  RyVelocityTargetSpecify=off  RyVelocityTargetPriority=High  RyVelocityTargetValue=0  RyVelocityTargetValueUnits=deg/s  RyEquilibriumPosition=0  RyEquilibriumPositionUnits=deg  RySpringStiffness=0  RySpringStiffnessUnits=N*m/deg  RyDampingCoefficient=0  RyDampingCoefficientUnits=N*m/(deg/s)  RyLowerLimitSpecify=off  RyLowerLimitBound=-90  RyLowerLimitBoundUnits=deg  RyLowerLimitStiffness=1e4  RyLowerLimitStiffnessUnits=N*m/deg  RyLowerLimitDamping=10  RyLowerLimitDampingUnits=N*m/(deg/s)  RyLowerLimitTransitionRegionWidth=0.1  RyLowerLimitTransitionRegionWidthUnits=deg  RyUpperLimitSpecify=off  RyUpperLimitBound=90  RyUpperLimitBoundUnits=deg  RyUpperLimitStiffness=1e4  RyUpperLimitStiffnessUnits=N*m/deg  RyUpperLimitDamping=10  RyUpperLimitDampingUnits=N*m/(deg/s)  RyUpperLimitTransitionRegionWidth=0.1  RyUpperLimitTransitionRegionWidthUnits=deg  RyTorqueActuationMode=NoTorque  RyMotionActuationMode=ComputedMotion  RySensePosition=off  RySenseVelocity=off  RySenseAcceleration=off  RySenseTorqueForce=off  RySenseLowerLimitTorqueForce=off  RySenseUpperLimitTorqueForce=off
  ChassisToLeftBoomCyl : sm_lib/Joints/Universal Joint  JointMode=Normal  CompositeWrenchDir=FollowerOnBase  CompositeWrenchFrame=BaseFrame  SenseConstraintForce=off  SenseConstraintTorque=off  SenseTotalForce=off  SenseTotalTorque=off  RxPositionTargetSpecify=off  RxPositionTargetPriority=High  RxPositionTargetValue=0  RxPositionTargetValueUnits=deg  RxVelocityTargetSpecify=off  RxVelocityTargetPriority=High  RxVelocityTargetValue=0  RxVelocityTargetValueUnits=deg/s  RxEquilibriumPosition=0  RxEquilibriumPositionUnits=deg  RxSpringStiffness=0  RxSpringStiffnessUnits=N*m/deg  RxDampingCoefficient=0  RxDampingCoefficientUnits=N*m/(deg/s)  RxLowerLimitSpecify=off  RxLowerLimitBound=-90  RxLowerLimitBoundUnits=deg  RxLowerLimitStiffness=1e4  RxLowerLimitStiffnessUnits=N*m/deg  RxLowerLimitDamping=10  RxLowerLimitDampingUnits=N*m/(deg/s)  RxLowerLimitTransitionRegionWidth=0.1  RxLowerLimitTransitionRegionWidthUnits=deg  RxUpperLimitSpecify=off  RxUpperLimitBound=90  RxUpperLimitBoundUnits=deg  RxUpperLimitStiffness=1e4  RxUpperLimitStiffnessUnits=N*m/deg  RxUpperLimitDamping=10  RxUpperLimitDampingUnits=N*m/(deg/s)  RxUpperLimitTransitionRegionWidth=0.1  RxUpperLimitTransitionRegionWidthUnits=deg  RxTorqueActuationMode=NoTorque  RxMotionActuationMode=ComputedMotion  RxSensePosition=off  RxSenseVelocity=off  RxSenseAcceleration=off  RxSenseTorqueForce=off  RxSenseLowerLimitTorqueForce=off  RxSenseUpperLimitTorqueForce=off  RyPositionTargetSpecify=off  RyPositionTargetPriority=High  RyPositionTargetValue=0  RyPositionTargetValueUnits=deg  RyVelocityTargetSpecify=off  RyVelocityTargetPriority=High  RyVelocityTargetValue=0  RyVelocityTargetValueUnits=deg/s  RyEquilibriumPosition=0  RyEquilibriumPositionUnits=deg  RySpringStiffness=0  RySpringStiffnessUnits=N*m/deg  RyDampingCoefficient=0  RyDampingCoefficientUnits=N*m/(deg/s)  RyLowerLimitSpecify=off  RyLowerLimitBound=-90  RyLowerLimitBoundUnits=deg  RyLowerLimitStiffness=1e4  RyLowerLimitStiffnessUnits=N*m/deg  RyLowerLimitDamping=10  RyLowerLimitDampingUnits=N*m/(deg/s)  RyLowerLimitTransitionRegionWidth=0.1  RyLowerLimitTransitionRegionWidthUnits=deg  RyUpperLimitSpecify=off  RyUpperLimitBound=90  RyUpperLimitBoundUnits=deg  RyUpperLimitStiffness=1e4  RyUpperLimitStiffnessUnits=N*m/deg  RyUpperLimitDamping=10  RyUpperLimitDampingUnits=N*m/(deg/s)  RyUpperLimitTransitionRegionWidth=0.1  RyUpperLimitTransitionRegionWidthUnits=deg  RyTorqueActuationMode=NoTorque  RyMotionActuationMode=ComputedMotion  RySensePosition=off  RySenseVelocity=off  RySenseAcceleration=off  RySenseTorqueForce=off  RySenseLowerLimitTorqueForce=off  RySenseUpperLimitTorqueForce=off
  LeftBoomCylToLeftBoomPiston : Subsystem  Tag=020d177e-0dad-473d-ac20-6fcc1e17d1fc
  pz : PMIOPort  Side=Left
  B : PMIOPort  Port=2  Side=Left
  F : PMIOPort  Port=3  Side=Right
  m : Outport
  wires:
  LeftBoomCylToLeftBoomPiston/1(m) -> m/1
  connections:
  BoomToLeftBoomPiston/LConn1 -- F/RConn1
  ChassisToLeftBoomCyl/RConn1 -- BoomLeftCyl/LConn1
  BoomToLeftBoomPiston/RConn1 -- BoomLeftPiston/RConn1
  BoomLeftCyl/RConn1 -- LeftBoomCylToLeftBoomPiston/LConn2
  B/RConn1 -- ChassisToLeftBoomCyl/LConn1
  LeftBoomCylToLeftBoomPiston/RConn1 -- BoomLeftPiston/LConn1
  pz/RConn1 -- LeftBoomCylToLeftBoomPiston/LConn1

== system Excavator_Motion/Excavator/Machine/Boom Cyl R ==
  BoomRightCyl : Subsystem  Tag=807666EC-A6D7-8B4A-99F9-B3248F920B99
  BoomRightPiston : Subsystem  Tag=00EE293A-0F1A-9247-9056-19EF67FE5161
  BoomToRightBoomPiston : sm_lib/Joints/Universal Joint  JointMode=Normal  CompositeWrenchDir=FollowerOnBase  CompositeWrenchFrame=BaseFrame  SenseConstraintForce=off  SenseConstraintTorque=off  SenseTotalForce=off  SenseTotalTorque=off  RxPositionTargetSpecify=off  RxPositionTargetPriority=High  RxPositionTargetValue=0  RxPositionTargetValueUnits=deg  RxVelocityTargetSpecify=off  RxVelocityTargetPriority=High  RxVelocityTargetValue=0  RxVelocityTargetValueUnits=deg/s  RxEquilibriumPosition=0  RxEquilibriumPositionUnits=deg  RxSpringStiffness=0  RxSpringStiffnessUnits=N*m/deg  RxDampingCoefficient=0  RxDampingCoefficientUnits=N*m/(deg/s)  RxLowerLimitSpecify=off  RxLowerLimitBound=-90  RxLowerLimitBoundUnits=deg  RxLowerLimitStiffness=1e4  RxLowerLimitStiffnessUnits=N*m/deg  RxLowerLimitDamping=10  RxLowerLimitDampingUnits=N*m/(deg/s)  RxLowerLimitTransitionRegionWidth=0.1  RxLowerLimitTransitionRegionWidthUnits=deg  RxUpperLimitSpecify=off  RxUpperLimitBound=90  RxUpperLimitBoundUnits=deg  RxUpperLimitStiffness=1e4  RxUpperLimitStiffnessUnits=N*m/deg  RxUpperLimitDamping=10  RxUpperLimitDampingUnits=N*m/(deg/s)  RxUpperLimitTransitionRegionWidth=0.1  RxUpperLimitTransitionRegionWidthUnits=deg  RxTorqueActuationMode=NoTorque  RxMotionActuationMode=ComputedMotion  RxSensePosition=off  RxSenseVelocity=off  RxSenseAcceleration=off  RxSenseTorqueForce=off  RxSenseLowerLimitTorqueForce=off  RxSenseUpperLimitTorqueForce=off  RyPositionTargetSpecify=off  RyPositionTargetPriority=High  RyPositionTargetValue=0  RyPositionTargetValueUnits=deg  RyVelocityTargetSpecify=off  RyVelocityTargetPriority=High  RyVelocityTargetValue=0  RyVelocityTargetValueUnits=deg/s  RyEquilibriumPosition=0  RyEquilibriumPositionUnits=deg  RySpringStiffness=0  RySpringStiffnessUnits=N*m/deg  RyDampingCoefficient=0  RyDampingCoefficientUnits=N*m/(deg/s)  RyLowerLimitSpecify=off  RyLowerLimitBound=-90  RyLowerLimitBoundUnits=deg  RyLowerLimitStiffness=1e4  RyLowerLimitStiffnessUnits=N*m/deg  RyLowerLimitDamping=10  RyLowerLimitDampingUnits=N*m/(deg/s)  RyLowerLimitTransitionRegionWidth=0.1  RyLowerLimitTransitionRegionWidthUnits=deg  RyUpperLimitSpecify=off  RyUpperLimitBound=90  RyUpperLimitBoundUnits=deg  RyUpperLimitStiffness=1e4  RyUpperLimitStiffnessUnits=N*m/deg  RyUpperLimitDamping=10  RyUpperLimitDampingUnits=N*m/(deg/s)  RyUpperLimitTransitionRegionWidth=0.1  RyUpperLimitTransitionRegionWidthUnits=deg  RyTorqueActuationMode=NoTorque  RyMotionActuationMode=ComputedMotion  RySensePosition=off  RySenseVelocity=off  RySenseAcceleration=off  RySenseTorqueForce=off  RySenseLowerLimitTorqueForce=off  RySenseUpperLimitTorqueForce=off
  ChassisToRightBoomCyl : sm_lib/Joints/Universal Joint  JointMode=Normal  CompositeWrenchDir=FollowerOnBase  CompositeWrenchFrame=BaseFrame  SenseConstraintForce=off  SenseConstraintTorque=off  SenseTotalForce=off  SenseTotalTorque=off  RxPositionTargetSpecify=off  RxPositionTargetPriority=High  RxPositionTargetValue=0  RxPositionTargetValueUnits=deg  RxVelocityTargetSpecify=off  RxVelocityTargetPriority=High  RxVelocityTargetValue=0  RxVelocityTargetValueUnits=deg/s  RxEquilibriumPosition=0  RxEquilibriumPositionUnits=deg  RxSpringStiffness=0  RxSpringStiffnessUnits=N*m/deg  RxDampingCoefficient=0  RxDampingCoefficientUnits=N*m/(deg/s)  RxLowerLimitSpecify=off  RxLowerLimitBound=-90  RxLowerLimitBoundUnits=deg  RxLowerLimitStiffness=1e4  RxLowerLimitStiffnessUnits=N*m/deg  RxLowerLimitDamping=10  RxLowerLimitDampingUnits=N*m/(deg/s)  RxLowerLimitTransitionRegionWidth=0.1  RxLowerLimitTransitionRegionWidthUnits=deg  RxUpperLimitSpecify=off  RxUpperLimitBound=90  RxUpperLimitBoundUnits=deg  RxUpperLimitStiffness=1e4  RxUpperLimitStiffnessUnits=N*m/deg  RxUpperLimitDamping=10  RxUpperLimitDampingUnits=N*m/(deg/s)  RxUpperLimitTransitionRegionWidth=0.1  RxUpperLimitTransitionRegionWidthUnits=deg  RxTorqueActuationMode=NoTorque  RxMotionActuationMode=ComputedMotion  RxSensePosition=off  RxSenseVelocity=off  RxSenseAcceleration=off  RxSenseTorqueForce=off  RxSenseLowerLimitTorqueForce=off  RxSenseUpperLimitTorqueForce=off  RyPositionTargetSpecify=off  RyPositionTargetPriority=High  RyPositionTargetValue=0  RyPositionTargetValueUnits=deg  RyVelocityTargetSpecify=off  RyVelocityTargetPriority=High  RyVelocityTargetValue=0  RyVelocityTargetValueUnits=deg/s  RyEquilibriumPosition=0  RyEquilibriumPositionUnits=deg  RySpringStiffness=0  RySpringStiffnessUnits=N*m/deg  RyDampingCoefficient=0  RyDampingCoefficientUnits=N*m/(deg/s)  RyLowerLimitSpecify=off  RyLowerLimitBound=-90  RyLowerLimitBoundUnits=deg  RyLowerLimitStiffness=1e4  RyLowerLimitStiffnessUnits=N*m/deg  RyLowerLimitDamping=10  RyLowerLimitDampingUnits=N*m/(deg/s)  RyLowerLimitTransitionRegionWidth=0.1  RyLowerLimitTransitionRegionWidthUnits=deg  RyUpperLimitSpecify=off  RyUpperLimitBound=90  RyUpperLimitBoundUnits=deg  RyUpperLimitStiffness=1e4  RyUpperLimitStiffnessUnits=N*m/deg  RyUpperLimitDamping=10  RyUpperLimitDampingUnits=N*m/(deg/s)  RyUpperLimitTransitionRegionWidth=0.1  RyUpperLimitTransitionRegionWidthUnits=deg  RyTorqueActuationMode=NoTorque  RyMotionActuationMode=ComputedMotion  RySensePosition=off  RySenseVelocity=off  RySenseAcceleration=off  RySenseTorqueForce=off  RySenseLowerLimitTorqueForce=off  RySenseUpperLimitTorqueForce=off
  RightBoomCylToRightBoomPiston : Subsystem  Tag=f4b02144-fc21-4459-875a-429d4adb33c6
  F : PMIOPort  Side=Right
  B : PMIOPort  Port=2  Side=Left
  connections:
  ChassisToRightBoomCyl/LConn1 -- B/RConn1
  BoomToRightBoomPiston/RConn1 -- BoomRightPiston/RConn1
  RightBoomCylToRightBoomPiston/RConn1 -- BoomRightPiston/LConn1
  BoomRightCyl/LConn1 -- ChassisToRightBoomCyl/RConn1
  BoomRightCyl/RConn1 -- RightBoomCylToRightBoomPiston/LConn1
  BoomToRightBoomPiston/LConn1 -- F/RConn1

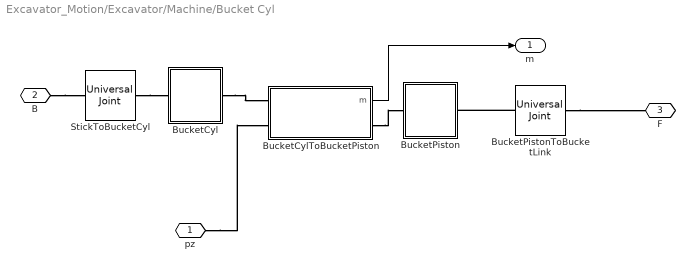
== system Excavator_Motion/Excavator/Machine/Bucket Cyl ==
  BucketCyl : Subsystem  Tag=9FAF18D5-1596-3A48-9F24-977D2E18A318
  BucketCylToBucketPiston : Subsystem  Tag=47fb7853-569f-437e-8d3d-7cddda445dda
  BucketPiston : Subsystem  Tag=EF45ED1F-ED8A-8D4B-830B-367867E4E96A
  BucketPistonToBucketLink : sm_lib/Joints/Universal Joint  JointMode=Normal  CompositeWrenchDir=FollowerOnBase  CompositeWrenchFrame=BaseFrame  SenseConstraintForce=off  SenseConstraintTorque=off  SenseTotalForce=off  SenseTotalTorque=off  RxPositionTargetSpecify=off  RxPositionTargetPriority=High  RxPositionTargetValue=0  RxPositionTargetValueUnits=deg  RxVelocityTargetSpecify=off  RxVelocityTargetPriority=High  RxVelocityTargetValue=0  RxVelocityTargetValueUnits=deg/s  RxEquilibriumPosition=0  RxEquilibriumPositionUnits=deg  RxSpringStiffness=0  RxSpringStiffnessUnits=N*m/deg  RxDampingCoefficient=0  RxDampingCoefficientUnits=N*m/(deg/s)  RxLowerLimitSpecify=off  RxLowerLimitBound=-90  RxLowerLimitBoundUnits=deg  RxLowerLimitStiffness=1e4  RxLowerLimitStiffnessUnits=N*m/deg  RxLowerLimitDamping=10  RxLowerLimitDampingUnits=N*m/(deg/s)  RxLowerLimitTransitionRegionWidth=0.1  RxLowerLimitTransitionRegionWidthUnits=deg  RxUpperLimitSpecify=off  RxUpperLimitBound=90  RxUpperLimitBoundUnits=deg  RxUpperLimitStiffness=1e4  RxUpperLimitStiffnessUnits=N*m/deg  RxUpperLimitDamping=10  RxUpperLimitDampingUnits=N*m/(deg/s)  RxUpperLimitTransitionRegionWidth=0.1  RxUpperLimitTransitionRegionWidthUnits=deg  RxTorqueActuationMode=NoTorque  RxMotionActuationMode=ComputedMotion  RxSensePosition=off  RxSenseVelocity=off  RxSenseAcceleration=off  RxSenseTorqueForce=off  RxSenseLowerLimitTorqueForce=off  RxSenseUpperLimitTorqueForce=off  RyPositionTargetSpecify=off  RyPositionTargetPriority=High  RyPositionTargetValue=0  RyPositionTargetValueUnits=deg  RyVelocityTargetSpecify=off  RyVelocityTargetPriority=High  RyVelocityTargetValue=0  RyVelocityTargetValueUnits=deg/s  RyEquilibriumPosition=0  RyEquilibriumPositionUnits=deg  RySpringStiffness=0  RySpringStiffnessUnits=N*m/deg  RyDampingCoefficient=0  RyDampingCoefficientUnits=N*m/(deg/s)  RyLowerLimitSpecify=off  RyLowerLimitBound=-90  RyLowerLimitBoundUnits=deg  RyLowerLimitStiffness=1e4  RyLowerLimitStiffnessUnits=N*m/deg  RyLowerLimitDamping=10  RyLowerLimitDampingUnits=N*m/(deg/s)  RyLowerLimitTransitionRegionWidth=0.1  RyLowerLimitTransitionRegionWidthUnits=deg  RyUpperLimitSpecify=off  RyUpperLimitBound=90  RyUpperLimitBoundUnits=deg  RyUpperLimitStiffness=1e4  RyUpperLimitStiffnessUnits=N*m/deg  RyUpperLimitDamping=10  RyUpperLimitDampingUnits=N*m/(deg/s)  RyUpperLimitTransitionRegionWidth=0.1  RyUpperLimitTransitionRegionWidthUnits=deg  RyTorqueActuationMode=NoTorque  RyMotionActuationMode=ComputedMotion  RySensePosition=off  RySenseVelocity=off  RySenseAcceleration=off  RySenseTorqueForce=off  RySenseLowerLimitTorqueForce=off  RySenseUpperLimitTorqueForce=off
  StickToBucketCyl : sm_lib/Joints/Universal Joint  JointMode=Normal  CompositeWrenchDir=FollowerOnBase  CompositeWrenchFrame=BaseFrame  SenseConstraintForce=off  SenseConstraintTorque=off  SenseTotalForce=off  SenseTotalTorque=off  RxPositionTargetSpecify=off  RxPositionTargetPriority=High  RxPositionTargetValue=0  RxPositionTargetValueUnits=deg  RxVelocityTargetSpecify=off  RxVelocityTargetPriority=High  RxVelocityTargetValue=0  RxVelocityTargetValueUnits=deg/s  RxEquilibriumPosition=0  RxEquilibriumPositionUnits=deg  RxSpringStiffness=0  RxSpringStiffnessUnits=N*m/deg  RxDampingCoefficient=0  RxDampingCoefficientUnits=N*m/(deg/s)  RxLowerLimitSpecify=off  RxLowerLimitBound=-90  RxLowerLimitBoundUnits=deg  RxLowerLimitStiffness=1e4  RxLowerLimitStiffnessUnits=N*m/deg  RxLowerLimitDamping=10  RxLowerLimitDampingUnits=N*m/(deg/s)  RxLowerLimitTransitionRegionWidth=0.1  RxLowerLimitTransitionRegionWidthUnits=deg  RxUpperLimitSpecify=off  RxUpperLimitBound=90  RxUpperLimitBoundUnits=deg  RxUpperLimitStiffness=1e4  RxUpperLimitStiffnessUnits=N*m/deg  RxUpperLimitDamping=10  RxUpperLimitDampingUnits=N*m/(deg/s)  RxUpperLimitTransitionRegionWidth=0.1  RxUpperLimitTransitionRegionWidthUnits=deg  RxTorqueActuationMode=NoTorque  RxMotionActuationMode=ComputedMotion  RxSensePosition=off  RxSenseVelocity=off  RxSenseAcceleration=off  RxSenseTorqueForce=off  RxSenseLowerLimitTorqueForce=off  RxSenseUpperLimitTorqueForce=off  RyPositionTargetSpecify=off  RyPositionTargetPriority=High  RyPositionTargetValue=0  RyPositionTargetValueUnits=deg  RyVelocityTargetSpecify=off  RyVelocityTargetPriority=High  RyVelocityTargetValue=0  RyVelocityTargetValueUnits=deg/s  RyEquilibriumPosition=0  RyEquilibriumPositionUnits=deg  RySpringStiffness=0  RySpringStiffnessUnits=N*m/deg  RyDampingCoefficient=0  RyDampingCoefficientUnits=N*m/(deg/s)  RyLowerLimitSpecify=off  RyLowerLimitBound=-90  RyLowerLimitBoundUnits=deg  RyLowerLimitStiffness=1e4  RyLowerLimitStiffnessUnits=N*m/deg  RyLowerLimitDamping=10  RyLowerLimitDampingUnits=N*m/(deg/s)  RyLowerLimitTransitionRegionWidth=0.1  RyLowerLimitTransitionRegionWidthUnits=deg  RyUpperLimitSpecify=off  RyUpperLimitBound=90  RyUpperLimitBoundUnits=deg  RyUpperLimitStiffness=1e4  RyUpperLimitStiffnessUnits=N*m/deg  RyUpperLimitDamping=10  RyUpperLimitDampingUnits=N*m/(deg/s)  RyUpperLimitTransitionRegionWidth=0.1  RyUpperLimitTransitionRegionWidthUnits=deg  RyTorqueActuationMode=NoTorque  RyMotionActuationMode=ComputedMotion  RySensePosition=off  RySenseVelocity=off  RySenseAcceleration=off  RySenseTorqueForce=off  RySenseLowerLimitTorqueForce=off  RySenseUpperLimitTorqueForce=off
  pz : PMIOPort  Side=Left
  B : PMIOPort  Port=2  Side=Left
  F : PMIOPort  Port=3  Side=Right
  m : Outport
  wires:
  BucketCylToBucketPiston/1(m) -> m/1
  connections:
  BucketPistonToBucketLink/LConn1 -- BucketPiston/RConn1
  BucketCylToBucketPiston/RConn1 -- BucketPiston/LConn1
  StickToBucketCyl/RConn1 -- BucketCyl/LConn1
  BucketPistonToBucketLink/RConn1 -- F/RConn1
  BucketCyl/RConn1 -- BucketCylToBucketPiston/LConn1
  B/RConn1 -- StickToBucketCyl/LConn1
  pz/RConn1 -- BucketCylToBucketPiston/LConn2

== system Excavator_Motion/Excavator/Machine/BucketLoads ==
  qBucket : Inport
  BucketForces : sm_lib/Forces and Torques/External Force and Torque  EnableForceX=off  EnableForceY=on  EnableForceZ=on  EnableForce=off  ForceResolutionFrame=World  EnableTorqueX=off  EnableTorqueY=off  EnableTorqueZ=off  EnableTorque=off  TorqueResolutionFrame=AttachedFrame
  BucketLoadsVariant : Subsystem  Variant=on
  Bus Creator : BusCreator  Inputs=2
  Simulink-PS Converter : nesl_utility/Simulink-PS Converter  PhysicalDomain=network_engine_domain  SubClassName=ps_input  LeftPortType=input  RightPortType=output  PseudoPeriodic=off  Frequencies=[]  NoiseDistribution=none  NoiseParameters=[]  Unit=kN  AffineConversion=off  FilteringAndDerivatives=provide  SimscapeFilterOrder=1  InputFilterTimeConstant=0.001  UdotUserProvided=0
  Simulink-PS Converter1 : nesl_utility/Simulink-PS Converter  PhysicalDomain=network_engine_domain  SubClassName=ps_input  LeftPortType=input  RightPortType=output  PseudoPeriodic=off  Frequencies=[]  NoiseDistribution=none  NoiseParameters=[]  Unit=kN  AffineConversion=off  FilteringAndDerivatives=provide  SimscapeFilterOrder=1  InputFilterTimeConstant=0.001  UdotUserProvided=0
  Terminator : Terminator
  Frc : PMIOPort  Side=Right
  wires:
  BucketLoadsVariant/1(BucketForceY) -> Bus Creator/1, Simulink-PS Converter/1  "fLong"
  BucketLoadsVariant/2(BucketForceZ) -> Bus Creator/2, Simulink-PS Converter1/1  "fVert"
  qBucket/1 -> BucketLoadsVariant/1(BucketAngle)
  Bus Creator/1 -> Terminator/1  "BucketSoilLoad"
  connections:
  BucketForces/RConn1 -- Frc/RConn1 -- BucketLoadsVariant/LConn1
  Simulink-PS Converter/RConn1 -- BucketForces/LConn1
  Simulink-PS Converter1/RConn1 -- BucketForces/LConn2

== system Excavator_Motion/Excavator/Machine/Gravity ==
  Constant : Constant  Value=0
  Constant1 : Constant  Value=0
  Constant2 : Constant  Value=gravity
  Integrator : Integrator  LimitOutput=on  UpperSaturationLimit=0  LowerSaturationLimit=gravity
  Mux : Mux  Inputs=3
  g : Outport
  wires:
  Constant1/1 -> Mux/1
  Integrator/1 -> Mux/3
  Constant/1 -> Mux/2
  Constant2/1 -> Integrator/1
  Mux/1 -> g/1
